simulink model "task2BPAM_22_110107589"  (R2023b)
settings: Solver=FixedStepAuto  StartTime=0.0  StopTime=4*8-1  RelTol=1e-3  EnableMultiTasking=on
libraries: commchan3 x1, simulink x1, dspsrcs4 x1, dspsigops x1
settings Model: LastModifiedBy=gowrav -local
settings SolverCC: AutoInsertRateTranBlk=on

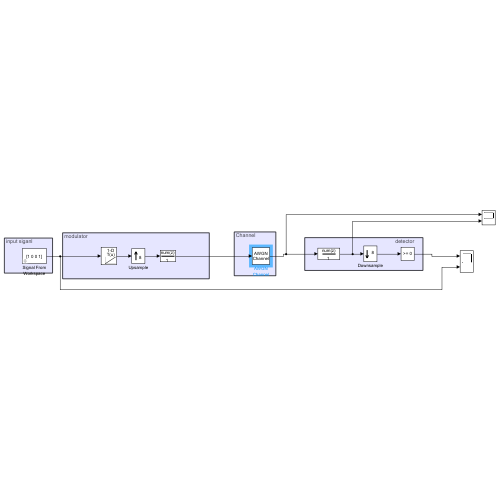
[thumbnail: Simulink's stored preview of the top-level diagram]
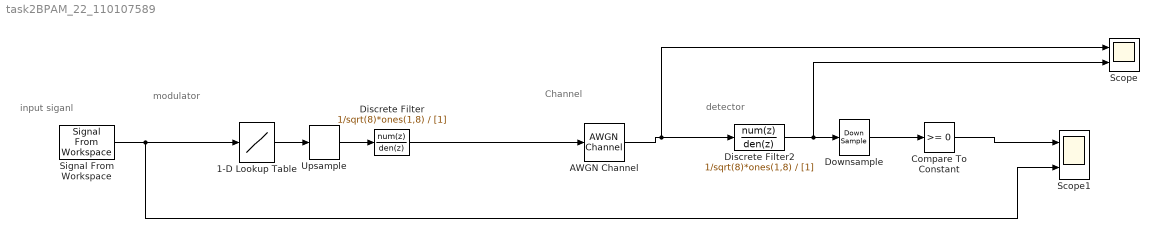
== system task2BPAM_22_110107589 ==
  note: detector
  note: Channel
  note: input siganl
  note: modulator
  1-D Lookup Table : Lookup_n-D  NumberOfTableDimensions=1  BreakpointsForDimension1=[0 1]  Table=[-1 1]  InternalRulePriority=Speed  RndMeth=Simplest
  AWGN Channel : commchan3/AWGN Channel  LegacyMode=on  NoiseMethod="Signal to noise ratio  (SNR)"  noiseMode="Signal to noise ratio  (Es/No)"  EbNo=10  EsNo=40  SNR=10  BitsPerSymbol=1  SignalPower=1  SamplesPerSymbol=1  SymbolPeriod=1  VarianceSource=Parameter  Variance=1  RandomStream=Global stream  Seed=110107589  SimulateUsing=Code generation
  Compare To Constant : simulink/Logic and Bit Operations/Compare To Constant  relop=>=  const=0  OutDataTypeStr=boolean
  Discrete Filter : DiscreteFilter  Numerator=1/sqrt(8)*ones(1,8)  Denominator=[1]
  Discrete Filter2 : DiscreteFilter  Numerator=1/sqrt(8)*ones(1,8)  Denominator=[1]
  Downsample : DownSample  N=8  RateOptions=Allow multirate processing
  Scope : Scope  NumInputPorts=2
  Scope1 : Scope  NumInputPorts=2
  Signal From Workspace : dspsrcs4/Signal From Workspace  X=[1 0 0 1]  Ts=8  nsamps=1  OutputAfterFinalValue=Setting to zero  ignoreOrWarnInputAndFrameLengths=off  OutputFrames=off
  Upsample : dspsigops/Upsample  FactorSource=Dialog parameter  N=8  Nmax=16  phase=0  RateOptions=Allow multirate processing  ic=0  mode=Unused parameter value
      settings: LibrarySourceBlock=dsphdlsupportsigops/Upsample
  wires:
  Signal From Workspace/1 -> Scope1/2, 1-D Lookup Table/1
  1-D Lookup Table/1 -> Upsample/1
  Upsample/1 -> Discrete Filter/1
  Discrete Filter/1 -> AWGN Channel/1
  AWGN Channel/1 -> Scope/1, Discrete Filter2/1
  Downsample/1 -> Compare To Constant/1
  Compare To Constant/1 -> Scope1/1
  Discrete Filter2/1 -> Downsample/1, Scope/2
